simulink model "controlAerobi"  (R2017b)
settings: Solver=FixedStepDiscrete  StartTime=0.0  StopTime=inf  FixedStep=Ts  RelTol=1e-3
InitFcn:
  | load Navio2_bus;
  | Ts=0.0025;
StopFcn:
  | %save_system('controlAerobi.slx');
  | %run('D:\Eclipse_Workspaces\workspace_rasp\AutoPilot\contAerobi\UpdateFiles\CopyBuildFiles.m');
undefined symbols (not defined in the file or in its folder): DiscIntNeverNeededParam
libraries: simulink x36, sharedutil x1, sharedtransform x1, dspsigops x1
(part 1 of 4)
CloseFcn:
  | %save_system('controlAerobi.slx');
settings Model: SimulationMode=external  ExtModeTrigDuration=400000  ExtModeArchiveFileName=apAerobi  ExtModeArchiveDirName=/home/ae-grvc/Documentos/Workspace/AutoPilot/GRVCAutopilot/Logs  ExtModeLogAll=off  Creator=GRVC  LastModifiedBy=root
settings SolverCC: PositivePriorityOrder=on
settings DataIOCC: SaveFormat=Array  SaveOutput=off  SaveTime=off
settings OptimizationCC: MemcpyThreshold=128  EfficientFloat2IntCast=on  MaxStackSize=128
settings DebuggingCC: SolverPrmCheckMsg=warning  IntegerOverflowMsg=none  ParameterTunabilityLossMsg=error  InvalidFcnCallConnMsg=warning  FcnCallInpInsideContextMsg=warning  BusObjectLabelMismatch=error  RootOutportRequireBusObject=error  ModelReferenceIOMsg=error  ModelReferenceIOMismatchMessage=error  ModelReferenceDataLoggingMessage=error  StateNameClashWarn=warning  SFUnexpectedBacktrackingDiag=warning  SFNoUnconditionalDefaultTransitionDiag=warning  SFExecutionAtInitializationDiag=none  IntegerSaturationMsg=none
settings HardwareCC: ProdBitPerPointer=32  ProdBitPerSizeT=32  ProdBitPerPtrDiffT=32  ProdLargestAtomicInteger=Long  ProdLargestAtomicFloat=Double  ProdWordSize=32  ProdHWDeviceType=ARM Compatible->ARM Cortex
settings ModelReferenceCC: ModelReferenceNumInstancesAllowed=Single  ModelReferencePassRootInputsByReference=off  PropagateSignalLabelsOutOfModel=off
settings SFSimCC: SimParseCustomCode=off  MATLABDynamicMemAlloc=off
settings RTWCC: SystemTargetFile=ert.tlc  HardwareBoard=Raspberry Pi  TemplateMakefile=ert_default_tmf  GenerateReport=on  RTWVerbose=off  CustomInclude=/home/ae-grvc/Documentos/Workspace/libshm_navio  Toolchain=GNU GCC Raspberry Pi  BuildConfiguration=Faster Runs  IncludeHyperlinkInReport=on  TargetLang=C++  GenerateTraceInfo=on  GenerateTraceReport=on  GenerateTraceReportSl=on  GenerateTraceReportSf=on  GenerateTraceReportEml=on
settings RTWCC: CustomHeaderCode=|
  | #include <shm_util.h>
  | #include <shm_channels.h>
settings CodeAppCC: ForceParamTrailComments=on  IgnoreCustomStorageClasses=off  CustomSymbolStrType=$N$R$M  StateflowObjectComments=on  InternalIdentifier=Classic
settings ERTTargetCC: UtilityFuncGeneration=Shared location  MatFileLogging=on  SupportComplex=off  SupportVariableSizeSignals=on  ExtMode=on  ExtModeMexArgs='navioAE-1.local' 0 17725 5  ConvertIfToSwitch=off  SuppressUnreachableDefaultCases=off  EnableUserReplacementTypes=on  MemSecPackage=Simulink  MemSecDataConstants=MemConst

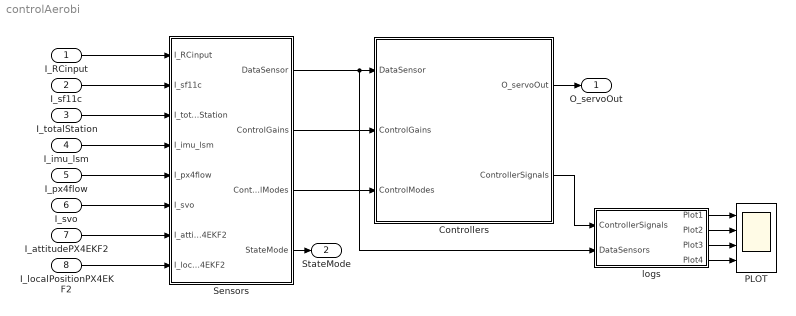
== system controlAerobi ==
  I_RCinput : Inport  OutDataTypeStr=Bus: shm_RCin
  I_sf11c : Inport  Port=2  OutDataTypeStr=Bus: shm_lightware
  I_totalStation : Inport  Port=3  OutDataTypeStr=Bus: shm_totalStation
  I_imu_lsm : Inport  Port=4  OutDataTypeStr=Bus: shm_imu
  I_px4flow : Inport  Port=5  OutDataTypeStr=Bus: shm_px4flow
  I_svo : Inport  Port=6  OutDataTypeStr=Bus: shm_svo
  I_attitudePX4EKF2 : Inport  Port=7  OutDataTypeStr=Bus: shm_attitudePX4EKF2
  I_localPositionPX4EKF2 : Inport  Port=8  OutDataTypeStr=Bus: shm_localPositionPX4EKF2
  Controllers : Subsystem
  PLOT : Scope  NumInputPorts=4
  Sensors : Subsystem
  logs : Subsystem  mask(Select signals to plot){SelectPlot1=roll, SelectPlot2=pitch, SelectPlot3=yaw, SelectPlot4=dyaw}
      mask prompts: SelectPlot1 "Select First Plot"; SelectPlot2 "Select Second Plot"; SelectPlot3 "Select Third Plot"; SelectPlot4 "Select Fourth Plot"
      mask TypeOptions SelectPlot1: roll | pitch | yaw | droll | dpitch | dyaw | x | y | z | dx | dy | dz | Rotors 1 & 2 | Rotors 3 & 4
      mask TypeOptions SelectPlot2: roll | pitch | yaw | droll | dpitch | dyaw | x | y | z | dx | dy | dz | Rotors 1 & 2 | Rotors 3 & 4
      mask TypeOptions SelectPlot3: roll | pitch | yaw | droll | dpitch | dyaw | x | y | z | dx | dy | dz | Rotors 1 & 2 | Rotors 3 & 4
      mask TypeOptions SelectPlot4: roll | pitch | yaw | droll | dpitch | dyaw | x | y | z | dx | dy | dz | Rotors 1 & 2 | Rotors 3 & 4
  O_servoOut : Outport  OutDataTypeStr=Bus: shm_RCou
  StateMode : Outport  Port=2
  wires:
  Sensors/2(ControlGains) -> Controllers/2(ControlGains)
  Sensors/3(ControlModes) -> Controllers/3(ControlModes)
  Controllers/1(O_servoOut) -> O_servoOut/1
  I_imu_lsm/1 -> Sensors/4(I_imu_lsm)
  logs/3(Plot3) -> PLOT/3
  I_px4flow/1 -> Sensors/5(I_px4flow)
  logs/4(Plot4) -> PLOT/4
  I_totalStation/1 -> Sensors/3(I_totalStation)
  logs/2(Plot2) -> PLOT/2
  Sensors/1(DataSensor) -> logs/2(DataSensors), Controllers/1(DataSensor)
  I_sf11c/1 -> Sensors/2(I_sf11c)
  Controllers/2(ControllerSignals) -> logs/1(ControllerSignals)
  Sensors/4(StateMode) -> StateMode/1
  logs/1(Plot1) -> PLOT/1
  I_RCinput/1 -> Sensors/1(I_RCinput)
  I_svo/1 -> Sensors/6(I_svo)
  I_attitudePX4EKF2/1 -> Sensors/7(I_attitudePX4EKF2)
  I_localPositionPX4EKF2/1 -> Sensors/8(I_localPositionPX4EKF2)

== system controlAerobi/Controllers ==
  DataSensor : Inport
  ControlGains : Inport  Port=2
  ControlModes : Inport  Port=3
  Quadrotor_Controllers : Subsystem
  O_servoOut : Outport  OutDataTypeStr=Bus: shm_RCou
  ControllerSignals : Outport  Port=2
  wires:
  DataSensor/1 -> Quadrotor_Controllers/1(DataSensor)
  Quadrotor_Controllers/1(ControllerSignals) -> ControllerSignals/1
  Quadrotor_Controllers/2(O_servoOut) -> O_servoOut/1
  ControlModes/1 -> Quadrotor_Controllers/3(ControlModes)
  ControlGains/1 -> Quadrotor_Controllers/2(ControlGains)

== system controlAerobi/Sensors ==
  I_RCinput : Inport  OutDataTypeStr=Bus: shm_RCin
  I_sf11c : Inport  Port=2  OutDataTypeStr=Bus: shm_lightware
  I_totalStation : Inport  Port=3  OutDataTypeStr=Bus: shm_totalStation
  I_imu_lsm : Inport  Port=4  OutDataTypeStr=Bus: shm_imu
  I_px4flow : Inport  Port=5  OutDataTypeStr=Bus: shm_px4flow
  I_svo : Inport  Port=6  OutDataTypeStr=Bus: shm_svo
  I_attitudePX4EKF2 : Inport  Port=7  OutDataTypeStr=Bus: shm_attitudePX4EKF2
  I_localPositionPX4EKF2 : Inport  Port=8  OutDataTypeStr=Bus: shm_localPositionPX4EKF2
  Bus Creator : BusCreator  Inputs=3
  Bus Creator1 : BusCreator  Inputs=2
  Geometric_Control_gains : Subsystem
  PID_cascade_gains : Subsystem
  RadioChannels : Subsystem
  ViewFlightMode : Subsystem
  attitude : Subsystem
  control_modes : Subsystem
  position : Subsystem
  DataSensor : Outport
  ControlGains : Outport  Port=2
  ControlModes : Outport  Port=3
  StateMode : Outport  Port=4
  wires:
  position/1(position_) -> Bus Creator/2  "position_"
  RadioChannels/1(Channels) -> Bus Creator/3  "channels"
  attitude/1(attitude_) -> position/1(attitude_), Bus Creator/1  "attitude_"
  I_RCinput/1 -> RadioChannels/1(I_RCinput)
  I_sf11c/1 -> position/2(I_sf11c)
  I_totalStation/1 -> position/3(I_totalStation)
  I_imu_lsm/1 -> attitude/1(I_imu_lsm)
  Bus Creator/1 -> control_modes/1(DataSensors), DataSensor/1
  PID_cascade_gains/1(PIDControlGains) -> Bus Creator1/1  "PIDgains"
  Geometric_Control_gains/1(GeometricControlGains) -> Bus Creator1/2  "GeometricGains"
  Bus Creator1/1 -> ControlGains/1
  control_modes/1(controlModes) -> position/6(ControlModes), ViewFlightMode/1(ControlModes), ControlModes/1
  ViewFlightMode/1(StateMode) -> StateMode/1
  I_px4flow/1 -> position/4(I_px4flow)
  I_svo/1 -> position/5(I_svo)
  I_attitudePX4EKF2/1 -> attitude/2(I_attitudePX4EKF2)
  I_localPositionPX4EKF2/1 -> position/7(I_localPositionPX4EKF2)

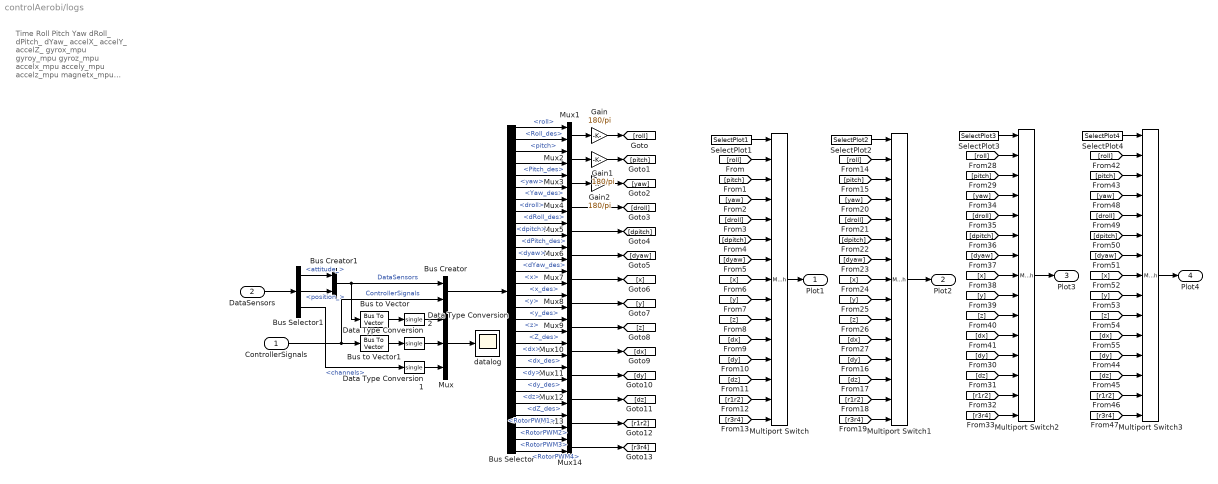
== system controlAerobi/logs ==
  note: Time
      | Roll
      | Pitch
      | Yaw
      | dRoll_
      | dPitch_
      | dYaw_
      | accelX_
      | accelY_
      | accelZ_
      | gyrox_mpu
      | gyroy_mpu
      | gyroz_mpu
      | accelx_mpu
      | accely_mpu
      | accelz_mpu
      | magnetx_mpu
      | magnety_mpu
      | magentz_mpu
      | gyrox_lsm
      | gyroy_lsm
      | gyroz_lsm
      | accelx_lsm
      | accely_lsm
      | accelz_lsm
      | magnetx_lsm
      | magnety_lsm
      | magnetz_lsm
      | GPS_solution
      | x_
      | y_
      | z_
      | dx_
      | dy_
      | dz_
      | z_sf11c
      | x_totalStation
      | y_totalStation
      | z_totalStation
      | time_totalStation
      | x_des
      | y_des
      | dx_des
      | dy_des
      | thrust
      | z_des
      | dz_des
      | roll_des
      | pitch_des
      | yaw_des
      | droll_des
      | dpitch_des
      | dyaw_des
      | RotorPWM1
      | RotorPWM2
      | RotorPWM3
      | RotorPWM4
      | Channel1
      | Channel2
      | Channel3
      | Channel4
      | Channel5
      | Channel6
      | Channel7
      | Channel8
      | Channel9
      | Channel10
  ControllerSignals : Inport
  DataSensors : Inport  Port=2
  Bus Creator : BusCreator  Inputs=2
  Bus Creator1 : BusCreator  Inputs=2
  Bus Selector : BusSelector  OutputSignals=DataSensors.attitude_.AngularPosition.roll,ControllerSignals.ControllersSignalsDesired.AttitudeSignals.AngularPositionDes.Roll_des,DataSensors.attitude_.AngularPosition.pitch,ControllerSignals.ControllersSignalsDesired.AttitudeSignals.AngularPositionDes.Pitch_des,DataSensors.attitude_.AngularPosition.yaw,ControllerSignals.ControllersSignalsDesired.AttitudeSignals.AngularPositionDes.Yaw_des,DataSensors.attitude_.AngularRates.droll,ControllerSignals.ControllersSignalsDesired.AttitudeSignals.AngularRateDes.dRoll_des,DataSensors.attitude_.AngularRates.dpitch,ControllerSignals.ControllersSignalsDesired.AttitudeSignals.AngularRateDes.dPitch_des,DataSensors.attitude_.AngularRates.dyaw,ControllerSignals.ControllersSignalsDesired.AttitudeSignals.AngularRateDes.dYaw_des,DataSensors.position_.Position.x,ControllerSignals.ControllersSignalsDesired.PositionSignals.x_des,DataSensors.position_.Position.y,ControllerSignals.ControllersSignalsDesired.PositionSignals.y_des,DataSensors.position_.Position.z,ControllerSignals.ControllersSignalsDesired.AltitudeSignals.ZController.Z_des,DataSensors.position_.Velocity.dx,ControllerSignals.ControllersSignalsDesired.PositionSignals.dx_des,DataSensors.position_.Velocity.dy,ControllerSignals.ControllersSignalsDesired.PositionSignals.dy_des,DataSensors.position_.Velocity.dz,ControllerSignals.ControllersSignalsDesired.AltitudeSignals.ZController.dZ_des,ControllerSignals.MixerSignals.RotorPWMSignals.RotorPWM1,ControllerSignals.MixerSignals.RotorPWMSignals.RotorPWM2,ControllerSignals.MixerSignals.RotorPWMSignals.RotorPWM3,ControllerSignals.MixerSignals.RotorPWMSignals.RotorPWM4
  Bus Selector1 : BusSelector  OutputSignals=attitude_,position_,channels
  Bus to Vector : BusToVector
  Bus to Vector1 : BusToVector
  Data Type Conversion : DataTypeConversion  OutDataTypeStr=single
  Data Type Conversion1 : DataTypeConversion  OutDataTypeStr=single
  Data Type Conversion2 : DataTypeConversion  OutDataTypeStr=single
  Gain : Gain  Gain=180/pi
  Gain1 : Gain  Gain=180/pi
  Gain2 : Gain  Gain=180/pi
  Multiport Switch{,1..3} (4 alike) : MultiPortSwitch  Inputs=14
  Mux : Mux  Inputs=3
  Mux{1..14} (14 alike) : Mux  Inputs=2
  SelectPlot1 : Constant  Value=SelectPlot1
  SelectPlot2 : Constant  Value=SelectPlot2
  SelectPlot3 : Constant  Value=SelectPlot3
  SelectPlot4 : Constant  Value=SelectPlot4
  datalog : Scope
  Plot1 : Outport
  Plot2 : Outport  Port=2
  Plot3 : Outport  Port=3
  Plot4 : Outport  Port=4
  wires:
  ControllerSignals/1 -> Bus to Vector1/1, Bus Creator/2  "ControllerSignals"
  Mux/1 -> datalog/1
  Bus to Vector1/1 -> Data Type Conversion/1
  Bus Creator/1 -> Bus Selector/1
  Bus Selector/2 -> Mux1/2  "<Roll_des>"
  Bus Selector/1 -> Mux1/1  "<roll>"
  Bus Selector/3 -> Mux2/1  "<pitch>"
  Bus Selector/4 -> Mux2/2  "<Pitch_des>"
  Bus Selector/5 -> Mux3/1  "<yaw>"
  Bus Selector/6 -> Mux3/2  "<Yaw_des>"
  Bus Selector/8 -> Mux4/2  "<dRoll_des>"
  Bus Selector/7 -> Mux4/1  "<droll>"
  Bus Selector/9 -> Mux5/1  "<dpitch>"
  Bus Selector/10 -> Mux5/2  "<dPitch_des>"
  Bus Selector/12 -> Mux6/2  "<dYaw_des>"
  Bus Selector/11 -> Mux6/1  "<dyaw>"
  Bus Selector/13 -> Mux7/1  "<x>"
  Bus Selector/14 -> Mux7/2  "<x_des>"
  Bus Selector/15 -> Mux8/1  "<y>"
  Bus Selector/16 -> Mux8/2  "<y_des>"
  Bus Selector/17 -> Mux9/1  "<z>"
  Bus Selector/18 -> Mux9/2  "<Z_des>"
  Bus Selector/19 -> Mux10/1  "<dx>"
  Bus Selector/20 -> Mux10/2  "<dx_des>"
  Bus Selector/22 -> Mux11/2  "<dy_des>"
  Bus Selector/21 -> Mux11/1  "<dy>"
  Bus Selector/23 -> Mux12/1  "<dz>"
  Bus Selector/24 -> Mux12/2  "<dZ_des>"
  Bus Selector/25 -> Mux13/1  "<RotorPWM1>"
  Bus Selector/26 -> Mux13/2  "<RotorPWM2>"
  Bus Selector/27 -> Mux14/1  "<RotorPWM3>"
  Bus Selector/28 -> Mux14/2  "<RotorPWM4>"
  SelectPlot1/1 -> Multiport Switch/1
  Mux2/1 -> Gain1/1
  Mux3/1 -> Gain2/1
  Mux4/1 -> [droll]
  Mux5/1 -> [dpitch]
  Mux6/1 -> [dyaw]
  Mux7/1 -> [x]
  Mux8/1 -> [y]
  Mux9/1 -> [z]
  Mux10/1 -> [dx]
  Mux11/1 -> [dy]
  Mux12/1 -> [dz]
  [y] -> Multiport Switch/9
  [x] -> Multiport Switch/8
  [dpitch] -> Multiport Switch/6
  [dyaw] -> Multiport Switch/7
  [z] -> Multiport Switch/10
  [droll] -> Multiport Switch/5
  [dx] -> Multiport Switch/11
  [yaw] -> Multiport Switch/4
  [pitch] -> Multiport Switch/3
  [dz] -> Multiport Switch/13
  [dy] -> Multiport Switch/12
  [roll] -> Multiport Switch/2
  [r1r2] -> Multiport Switch/14
  [r3r4] -> Multiport Switch/15
  SelectPlot2/1 -> Multiport Switch1/1
  [y] -> Multiport Switch1/9
  [x] -> Multiport Switch1/8
  [dpitch] -> Multiport Switch1/6
  [dyaw] -> Multiport Switch1/7
  [z] -> Multiport Switch1/10
  [droll] -> Multiport Switch1/5
  [dx] -> Multiport Switch1/11
  [yaw] -> Multiport Switch1/4
  [pitch] -> Multiport Switch1/3
  [dz] -> Multiport Switch1/13
  [dy] -> Multiport Switch1/12
  [roll] -> Multiport Switch1/2
  [r1r2] -> Multiport Switch1/14
  [r3r4] -> Multiport Switch1/15
  SelectPlot3/1 -> Multiport Switch2/1
  [y] -> Multiport Switch2/9
  [x] -> Multiport Switch2/8
  [dpitch] -> Multiport Switch2/6
  [dyaw] -> Multiport Switch2/7
  [z] -> Multiport Switch2/10
  [droll] -> Multiport Switch2/5
  [dx] -> Multiport Switch2/11
  [yaw] -> Multiport Switch2/4
  [pitch] -> Multiport Switch2/3
  [dz] -> Multiport Switch2/13
  [dy] -> Multiport Switch2/12
  [roll] -> Multiport Switch2/2
  [r1r2] -> Multiport Switch2/14
  [r3r4] -> Multiport Switch2/15
  SelectPlot4/1 -> Multiport Switch3/1
  [y] -> Multiport Switch3/9
  [x] -> Multiport Switch3/8
  [dpitch] -> Multiport Switch3/6
  [dyaw] -> Multiport Switch3/7
  [z] -> Multiport Switch3/10
  [droll] -> Multiport Switch3/5
  [dx] -> Multiport Switch3/11
  [yaw] -> Multiport Switch3/4
  [pitch] -> Multiport Switch3/3
  [dz] -> Multiport Switch3/13
  [dy] -> Multiport Switch3/12
  [roll] -> Multiport Switch3/2
  [r1r2] -> Multiport Switch3/14
  [r3r4] -> Multiport Switch3/15
  Multiport Switch/1 -> Plot1/1
  Multiport Switch1/1 -> Plot2/1
  Multiport Switch2/1 -> Plot3/1
  Multiport Switch3/1 -> Plot4/1
  Mux1/1 -> Gain/1
  Gain/1 -> [roll]
  Gain1/1 -> [pitch]
  Gain2/1 -> [yaw]
  Data Type Conversion/1 -> Mux/2
  Bus to Vector/1 -> Data Type Conversion2/1
  Mux13/1 -> [r1r2]
  Mux14/1 -> [r3r4]
  DataSensors/1 -> Bus Selector1/1
  Bus Creator1/1 -> Bus to Vector/1, Bus Creator/1  "DataSensors"
  Bus Selector1/1 -> Bus Creator1/1  "<attitude_>"
  Bus Selector1/2 -> Bus Creator1/2  "<position_>"
  Bus Selector1/3 -> Data Type Conversion1/1  "<channels>"
  Data Type Conversion1/1 -> Mux/3
  Data Type Conversion2/1 -> Mux/1

== system controlAerobi/Controllers/Quadrotor_Controllers ==
  DataSensor : Inport
  ControlGains : Inport  Port=2
  ControlModes : Inport  Port=3
  Bus Creator : BusCreator  Inputs=2
  Geometric_controller : Subsystem
  PID_cascade_controllers : Subsystem
  mixer : Subsystem
  switch_controllers : Subsystem
  ControllerSignals : Outport
  O_servoOut : Outport  Port=2  OutDataTypeStr=Bus: shm_RCou
  wires:
  mixer/2(O_servoOut) -> O_servoOut/1
  Bus Creator/1 -> ControllerSignals/1
  mixer/1(MixerSignals) -> Bus Creator/2  "MixerSignals"
  ControlModes/1 -> switch_controllers/3(ControlModes), mixer/2(ControlModes), Geometric_controller/3(ControlModes), PID_cascade_controllers/2(ControlModes)
  DataSensor/1 -> Geometric_controller/1(DataSensor), PID_cascade_controllers/1(DataSensor)
  ControlGains/1 -> Geometric_controller/2(ControlGains), PID_cascade_controllers/3(ControlGains)
  PID_cascade_controllers/1(ControllersSignalsDesired) -> Bus Creator/1  "ControllersSignalsDesired"
  PID_cascade_controllers/2(U_PID) -> switch_controllers/1(U_PID)
  Geometric_controller/1(U_GeometricControl) -> switch_controllers/2(U_GeometricControl)
  switch_controllers/1(U) -> mixer/1(U)

== system controlAerobi/Sensors/Geometric_Control_gains ==
  Bus Creator1 : BusCreator  Inputs=4
  Bus Creator2 : BusCreator  Inputs=10
  Bus Creator3 : BusCreator  Inputs=2
  CTf : Constant  Value=0.0008
  J : Constant  Value=[0.08 0 0; 0 0.08 0; 0 0 0.14]
  Mass : Constant  Value=1.97
  c1 : Constant  Value=[0.8; 0.8; 0.8]
  c2 : Constant  Value=[3; 3; 3]
  d : Constant  Value=0.2675
  k_I : Constant  Value=[55; 55; 55]
  k_Omega : Constant  Value=[8; 8; 8]
  k_R : Constant  Value=[60; 60; 60]
  k_i : Constant  Value=[0; 0; 0]
  k_v : Constant  Value=[10; 10; 10]
  k_x : Constant  Value=[10; 10; 10]
  sat_P : Constant  Value=[inf; inf; inf]
  sat_R : Constant  Value=[inf; inf; inf]
  GeometricControlGains : Outport
  wires:
  J/1 -> Bus Creator1/1  "J"
  CTf/1 -> Bus Creator1/4  "CTf"
  Mass/1 -> Bus Creator1/2  "Mass"
  d/1 -> Bus Creator1/3  "d"
  Bus Creator1/1 -> Bus Creator3/1  "UAVparameters"
  Bus Creator2/1 -> Bus Creator3/2  "Gains"
  Bus Creator3/1 -> GeometricControlGains/1
  k_R/1 -> Bus Creator2/1  "k_R"
  k_Omega/1 -> Bus Creator2/2  "k_Omega"
  k_x/1 -> Bus Creator2/6  "k_x"
  k_v/1 -> Bus Creator2/7  "k_v"
  c2/1 -> Bus Creator2/4  "c2"
  sat_R/1 -> Bus Creator2/5  "sat_R"
  k_I/1 -> Bus Creator2/3  "k_I"
  k_i/1 -> Bus Creator2/8  "k_i"
  c1/1 -> Bus Creator2/9  "c1"
  sat_P/1 -> Bus Creator2/10  "sat_P"

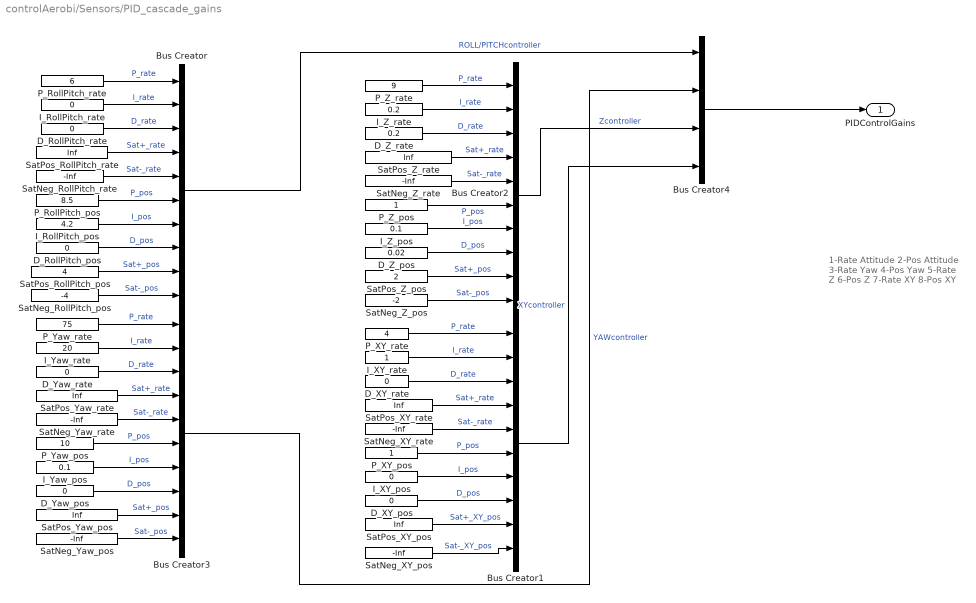
== system controlAerobi/Sensors/PID_cascade_gains ==
  note: 1-Rate Attitude
      | 2-Pos Attitude
      | 3-Rate Yaw
      | 4-Pos Yaw
      | 5-Rate Z
      | 6-Pos Z
      | 7-Rate XY
      | 8-Pos XY
  Bus Creator{,1..3} (4 alike) : BusCreator  Inputs=10
  Bus Creator4 : BusCreator  Inputs=4
  D_RollPitch_pos : Constant  Value=0
  D_RollPitch_rate : Constant  Value=0
  D_XY_pos : Constant  Value=0
  D_XY_rate : Constant  Value=0
  D_Yaw_pos : Constant  Value=0
  D_Yaw_rate : Constant  Value=0
  D_Z_pos : Constant  Value=0.02
  D_Z_rate : Constant  Value=0.2
  I_RollPitch_pos : Constant  Value=4.2
  I_RollPitch_rate : Constant  Value=0
  I_XY_pos : Constant  Value=0
  I_XY_rate : Constant
  I_Yaw_pos : Constant  Value=0.1
  I_Yaw_rate : Constant  Value=20
  I_Z_pos : Constant  Value=0.1
  I_Z_rate : Constant  Value=0.2
  P_RollPitch_pos : Constant  Value=8.5
  P_RollPitch_rate : Constant  Value=6
  P_XY_pos : Constant
  P_XY_rate : Constant  Value=4
  P_Yaw_pos : Constant  Value=10
  P_Yaw_rate : Constant  Value=75
  P_Z_pos : Constant
  P_Z_rate : Constant  Value=9
  SatNeg_RollPitch_pos : Constant  Value=-4
  SatNeg_RollPitch_rate : Constant  Value=-Inf
  SatNeg_XY_pos : Constant  Value=-Inf
  SatNeg_XY_rate : Constant  Value=-Inf
  SatNeg_Yaw_pos : Constant  Value=-Inf
  SatNeg_Yaw_rate : Constant  Value=-Inf
  SatNeg_Z_pos : Constant  Value=-2
  SatNeg_Z_rate : Constant  Value=-Inf
  SatPos_RollPitch_pos : Constant  Value=4
  SatPos_RollPitch_rate : Constant  Value=Inf
  SatPos_XY_pos : Constant  Value=Inf
  SatPos_XY_rate : Constant  Value=Inf
  SatPos_Yaw_pos : Constant  Value=Inf
  SatPos_Yaw_rate : Constant  Value=Inf
  SatPos_Z_pos : Constant  Value=2
  SatPos_Z_rate : Constant  Value=Inf
  PIDControlGains : Outport
  wires:
  SatPos_RollPitch_rate/1 -> Bus Creator/4  "Sat+_rate"
  D_RollPitch_rate/1 -> Bus Creator/3  "D_rate"
  P_RollPitch_rate/1 -> Bus Creator/1  "P_rate"
  I_RollPitch_rate/1 -> Bus Creator/2  "I_rate"
  SatNeg_RollPitch_rate/1 -> Bus Creator/5  "Sat-_rate"
  D_RollPitch_pos/1 -> Bus Creator/8  "D_pos"
  I_RollPitch_pos/1 -> Bus Creator/7  "I_pos"
  P_RollPitch_pos/1 -> Bus Creator/6  "P_pos"
  SatNeg_RollPitch_pos/1 -> Bus Creator/10  "Sat-_pos"
  SatPos_RollPitch_pos/1 -> Bus Creator/9  "Sat+_pos"
  SatPos_Yaw_rate/1 -> Bus Creator3/4  "Sat+_rate"
  SatNeg_Yaw_rate/1 -> Bus Creator3/5  "Sat-_rate"
  P_Yaw_rate/1 -> Bus Creator3/1  "P_rate"
  I_Yaw_rate/1 -> Bus Creator3/2  "I_rate"
  D_Yaw_rate/1 -> Bus Creator3/3  "D_rate"
  P_Yaw_pos/1 -> Bus Creator3/6  "P_pos"
  SatPos_Yaw_pos/1 -> Bus Creator3/9  "Sat+_pos"
  I_Yaw_pos/1 -> Bus Creator3/7  "I_pos"
  SatNeg_Yaw_pos/1 -> Bus Creator3/10  "Sat-_pos"
  D_Yaw_pos/1 -> Bus Creator3/8  "D_pos"
  SatPos_Z_rate/1 -> Bus Creator2/4  "Sat+_rate"
  SatNeg_Z_rate/1 -> Bus Creator2/5  "Sat-_rate"
  D_Z_rate/1 -> Bus Creator2/3  "D_rate"
  I_Z_rate/1 -> Bus Creator2/2  "I_rate"
  P_Z_rate/1 -> Bus Creator2/1  "P_rate"
  P_Z_pos/1 -> Bus Creator2/6  "P_pos"
  I_Z_pos/1 -> Bus Creator2/7  "I_pos"
  D_Z_pos/1 -> Bus Creator2/8  "D_pos"
  SatPos_Z_pos/1 -> Bus Creator2/9  "Sat+_pos"
  SatNeg_Z_pos/1 -> Bus Creator2/10  "Sat-_pos"
  SatPos_XY_rate/1 -> Bus Creator1/4  "Sat+_rate"
  SatNeg_XY_rate/1 -> Bus Creator1/5  "Sat-_rate"
  I_XY_rate/1 -> Bus Creator1/2  "I_rate"
  D_XY_rate/1 -> Bus Creator1/3  "D_rate"
  P_XY_rate/1 -> Bus Creator1/1  "P_rate"
  P_XY_pos/1 -> Bus Creator1/6  "P_pos"
  SatPos_XY_pos/1 -> Bus Creator1/9  "Sat+_XY_pos"
  SatNeg_XY_pos/1 -> Bus Creator1/10  "Sat-_XY_pos"
  I_XY_pos/1 -> Bus Creator1/7  "I_pos"
  Bus Creator/1 -> Bus Creator4/1  "ROLL/PITCHcontroller"
  Bus Creator3/1 -> Bus Creator4/2  "YAWcontroller"
  Bus Creator2/1 -> Bus Creator4/3  "Zcontroller"
  Bus Creator1/1 -> Bus Creator4/4  "XYcontroller"
  Bus Creator4/1 -> PIDControlGains/1
  D_XY_pos/1 -> Bus Creator1/8  "D_pos"

== system controlAerobi/Sensors/RadioChannels ==
  I_RCinput : Inport  OutDataTypeStr=Bus: shm_RCin
  Bus Selector2 : BusSelector  OutputSignals=_channel1,_channel2,_channel3,_channel4,_channel5,_channel6,_channel7,_channel8,_channel9,_channel10
  Mux1 : Mux  Inputs=10
  Channels : Outport
  wires:
  Bus Selector2/3 -> Mux1/3  "<_channel3>"
  Bus Selector2/4 -> Mux1/4  "<_channel4>"
  Bus Selector2/2 -> Mux1/2  "<_channel2>"
  Bus Selector2/5 -> Mux1/5  "<_channel5>"
  Bus Selector2/10 -> Mux1/10  "<_channel10>"
  Bus Selector2/1 -> Mux1/1  "<_channel1>"
  Bus Selector2/6 -> Mux1/6  "<_channel6>"
  Bus Selector2/7 -> Mux1/7  "<_channel7>"
  Bus Selector2/8 -> Mux1/8  "<_channel8>"
  Bus Selector2/9 -> Mux1/9  "<_channel9>"
  Mux1/1 -> Channels/1
  I_RCinput/1 -> Bus Selector2/1

== system controlAerobi/Sensors/ViewFlightMode ==
  ControlModes : Inport
  Bus Selector1 : BusSelector  OutputSignals=ModeControl.RESET,ModeControl.ALTHOLD,ModeControl.POS_HOLD
  Mux1 : Mux  Inputs=3
  State : Display
  StateMode : Outport
  wires:
  ControlModes/1 -> Bus Selector1/1
  Bus Selector1/2 -> Mux1/2  "<ALTHOLD>"
  Mux1/1 -> StateMode/1, State/1
  Bus Selector1/1 -> Mux1/1  "<RESET>"
  Bus Selector1/3 -> Mux1/3  "<POS_HOLD>"

== system controlAerobi/Sensors/attitude ==
  I_imu_lsm : Inport  OutDataTypeStr=Bus: shm_imu
  I_attitudePX4EKF2 : Inport  Port=2  OutDataTypeStr=Bus: shm_attitudePX4EKF2
  AttitudeEstimator : Subsystem
  Bus Creator2 : BusCreator  Inputs=4
  attitude_ : Outport
  wires:
  AttitudeEstimator/2(AnguraRates) -> Bus Creator2/2  "AngularRates"
  Bus Creator2/1 -> attitude_/1
  AttitudeEstimator/1(Attitude) -> Bus Creator2/1  "AngularPosition"
  AttitudeEstimator/3(Accelerometer) -> Bus Creator2/3  "Accelerometer"
  AttitudeEstimator/4(imuRaw) -> Bus Creator2/4  "imuRaw"
  I_imu_lsm/1 -> AttitudeEstimator/1(I_imu_lsm)
  I_attitudePX4EKF2/1 -> AttitudeEstimator/2(I_attitudePX4EKF2)

== system controlAerobi/Sensors/control_modes ==
  note: MODE:
      | 1.-ATTITUDE/RATE
      | 2.-ALT. HOLD
      | 3.-POS. HOLD
  DataSensors : Inport
  Bus Creator2 : BusCreator  Inputs=3
  ModeBlock : Subsystem
  PositionDesired : Subsystem
  Signals_to_references : Subsystem
  controlModes : Outport
  wires:
  Bus Creator2/1 -> controlModes/1
  DataSensors/1 -> Signals_to_references/1(uiPilotChannels), ModeBlock/1(Sticks)
  Signals_to_references/1(RemoteControl) -> Bus Creator2/1  "RemoteControl"
  ModeBlock/1(ModeControl) -> Bus Creator2/2  "ModeControl"
  PositionDesired/1(PositionDesired) -> Bus Creator2/3  "PositionDesired"

== system controlAerobi/Sensors/position ==
  attitude_ : Inport
  I_sf11c : Inport  Port=2  OutDataTypeStr=Bus: shm_lightware
  I_totalStation : Inport  Port=3  OutDataTypeStr=Bus: shm_totalStation
  I_px4flow : Inport  Port=4  OutDataTypeStr=Bus: shm_px4flow
  I_svo : Inport  Port=5  OutDataTypeStr=Bus: shm_svo
  ControlModes : Inport  Port=6
  I_localPositionPX4EKF2 : Inport  Port=7  OutDataTypeStr=Bus: shm_localPositionPX4EKF2
  Bus Creator2 : BusCreator  Inputs=4
  EKF_total_Station_Lidar : Subsystem
  GPS_px4 : Subsystem
  KQ : Constant  Value="[ 0 0.005  0 0.005  0 0.0025]"
  KR : Constant  Value=[0.01 0.1 0.01 0.1 0.05]
  PX4 : Scope
  SVO : Scope
  d_prism : Constant  Value=0.105
  d_sf11 : Constant  Value=0.048
  px4fow : Subsystem
  selector : Subsystem
  svo : Subsystem
  position_ : Outport
  wires:
  selector/1(GPS_Solution) -> Bus Creator2/1  "GPS_Solution"
  Bus Creator2/1 -> position_/1
  I_totalStation/1 -> EKF_total_Station_Lidar/1(I_totalStation), selector/1(I_totalStation)
  I_sf11c/1 -> EKF_total_Station_Lidar/2(I_sf11c)
  attitude_/1 -> EKF_total_Station_Lidar/3(attitude_), px4fow/1(attitude_)
  d_sf11/1 -> EKF_total_Station_Lidar/4(d_sf11)
  d_prism/1 -> EKF_total_Station_Lidar/5(d_prism)
  KQ/1 -> EKF_total_Station_Lidar/6(KQ)
  KR/1 -> EKF_total_Station_Lidar/7(KR)
  EKF_total_Station_Lidar/3(posRaw) -> Bus Creator2/4  "posRaw"
  selector/2(Position) -> Bus Creator2/2  "Position"
  selector/3(Velocity) -> Bus Creator2/3  "Velocity"
  GPS_px4/1(NED_position) -> selector/2(NED_pos_PX4)
  GPS_px4/2(NED_speed) -> selector/3(NED_vel_PX4)
  EKF_total_Station_Lidar/1(NED_position) -> selector/4(NED_pos_EKF)
  EKF_total_Station_Lidar/2(NED_speed) -> selector/5(NED_vel_EKF)
  ControlModes/1 -> px4fow/2(ControlModes), EKF_total_Station_Lidar/8(ControlModes)
  I_px4flow/1 -> px4fow/3(I_px4flow)
  px4fow/1(dxdyaxay) -> selector/6(NED_vel_PX4FLOW), PX4/1
  I_svo/1 -> svo/1(I_svo)
  svo/1(XYZ) -> SVO/1
  I_localPositionPX4EKF2/1 -> GPS_px4/1(I_localPositionPX4EKF2)

== system controlAerobi/Controllers/Quadrotor_Controllers/Geometric_controller ==
  DataSensor : Inport
  ControlGains : Inport  Port=2
  ControlModes : Inport  Port=3
  Bus Selector2 : BusSelector  OutputSignals=ModeControl.ALTHOLD,RemoteControl.Thrust/Zdes,ModeControl.RESET
  Mux : Mux
  Reset : Constant  Value=[0;0;0;0]
  Switch : Switch  Criteria=u2 ~= 0
  Switch1 : Switch  Criteria=u2 ~= 0
  attitude_tracking : Subsystem
  trajectory_tracking : Subsystem
  U_GeometricControl : Outport
  wires:
  Switch/1 -> U_GeometricControl/1
  Mux/1 -> Switch/1
  Reset/1 -> Switch/3
  DataSensor/1 -> trajectory_tracking/1(DataSensor), attitude_tracking/2(DataSensor)
  ControlGains/1 -> trajectory_tracking/2(ControlGains), attitude_tracking/3(ControlGains)
  ControlModes/1 -> trajectory_tracking/3(ControlModes), Bus Selector2/1, attitude_tracking/4(ControlModes)
  attitude_tracking/1(U2) -> Mux/2
  attitude_tracking/2(U3) -> Mux/3
  attitude_tracking/3(U4) -> Mux/4
  Switch1/1 -> Mux/1
  trajectory_tracking/1(f) -> Switch1/1
  Bus Selector2/2 -> Switch1/3  "<Thrust/Zdes>"
  trajectory_tracking/2(R_d_tracking) -> attitude_tracking/1(R_d_tracking)
  Bus Selector2/1 -> Switch1/2  "<ALTHOLD>"
  Bus Selector2/3 -> Switch/2  "<RESET>"

== system controlAerobi/Controllers/Quadrotor_Controllers/PID_cascade_controllers ==
  DataSensor : Inport
  ControlModes : Inport  Port=2
  ControlGains : Inport  Port=3
  Bus Creator1 : BusCreator  Inputs=3
  Mux : Mux
  PID_ATTITUDE_CONTROLLER : Subsystem
  PID_POSITION_CONTROLLER : Subsystem
  ControllersSignalsDesired : Outport
  U_PID : Outport  Port=2
  wires:
  ControlModes/1 -> PID_ATTITUDE_CONTROLLER/2(ControlModes), PID_POSITION_CONTROLLER/2(ControlModes)
  ControlGains/1 -> PID_ATTITUDE_CONTROLLER/3(ControlGains), PID_POSITION_CONTROLLER/3(ControlGains)
  DataSensor/1 -> PID_POSITION_CONTROLLER/1(DataSensor), PID_ATTITUDE_CONTROLLER/1(DataSensor)
  PID_POSITION_CONTROLLER/1(ref_att) -> PID_ATTITUDE_CONTROLLER/4(ref_att)
  PID_POSITION_CONTROLLER/4(U1) -> Mux/1  "U1"
  PID_ATTITUDE_CONTROLLER/3(U4) -> Mux/4  "U4"
  PID_ATTITUDE_CONTROLLER/2(U3) -> Mux/3  "U3"
  PID_ATTITUDE_CONTROLLER/1(U2) -> Mux/2  "U2"
  Mux/1 -> U_PID/1
  PID_POSITION_CONTROLLER/2(PositionSignals) -> Bus Creator1/1  "PositionSignals"
  PID_POSITION_CONTROLLER/3(AltitudeSignals) -> Bus Creator1/2  "AltitudeSignals"
  PID_ATTITUDE_CONTROLLER/4(AttitudeSignals) -> Bus Creator1/3  "AttitudeSignals"
  Bus Creator1/1 -> ControllersSignalsDesired/1

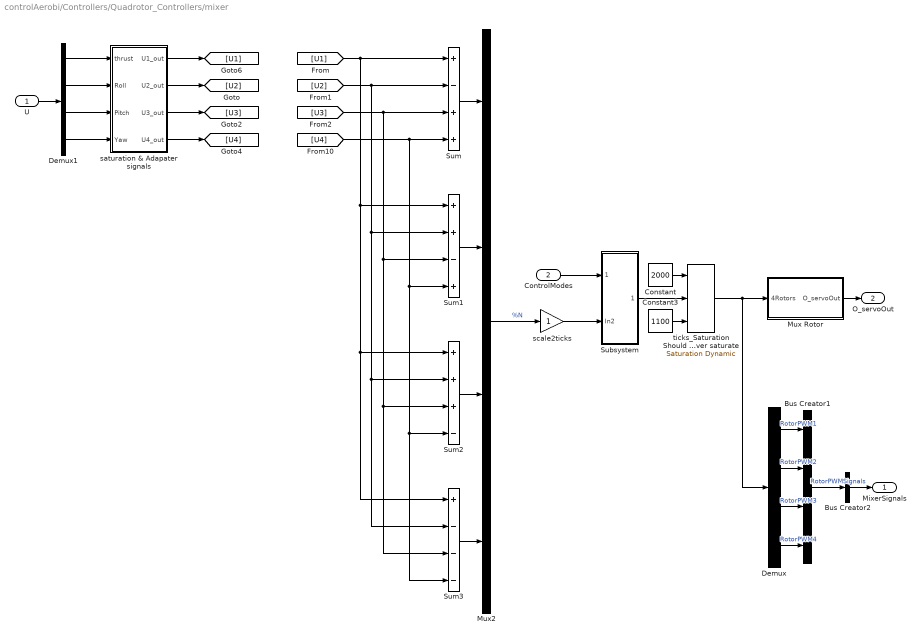
== system controlAerobi/Controllers/Quadrotor_Controllers/mixer ==
  U : Inport
  ControlModes : Inport  Port=2
  Bus Creator1 : BusCreator  Inputs=4
  Bus Creator2 : BusCreator  Inputs=1
  Constant : Constant  Value=2000
  Constant3 : Constant  Value=1100
  Demux : Demux
  Demux1 : Demux
  Mux Rotor : Subsystem
  Mux2 : Mux
  Subsystem : Subsystem
  Sum : Sum  Inputs=+-++
  Sum1 : Sum  Inputs=++-+
  Sum2 : Sum  Inputs=+++-
  Sum3 : Sum  Inputs=+---
  saturation & Adapater signals : Subsystem
  scale2ticks : Gain
  ticks_Saturation Should Never saturate : simulink/Discontinuities/Saturation Dynamic  OutMin=[]  OutMax=[]  OutDataTypeStr=Inherit: Same as second input  OutDataType=fixdt(1, 16)  OutScaling=2^-10  DoSatur=off
  MixerSignals : Outport
  O_servoOut : Outport  Port=2  OutDataTypeStr=Bus: shm_RCou
  wires:
  Constant3/1 -> ticks_Saturation Should Never saturate/3
  Constant/1 -> ticks_Saturation Should Never saturate/1
  Mux2/1 -> scale2ticks/1  "%N"
  Sum/1 -> Mux2/1
  Sum1/1 -> Mux2/2
  Sum3/1 -> Mux2/4
  ticks_Saturation Should Never saturate/1 -> Mux Rotor/1(4Rotors), Demux/1
  Sum2/1 -> Mux2/3
  saturation & Adapater signals/1(U1_out) -> [U1]
  saturation & Adapater signals/2(U2_out) -> [U2]
  saturation & Adapater signals/3(U3_out) -> [U3]
  Demux/1 -> Bus Creator1/1  "RotorPWM1"
  Demux/2 -> Bus Creator1/2  "RotorPWM2"
  Demux/3 -> Bus Creator1/3  "RotorPWM3"
  Demux/4 -> Bus Creator1/4  "RotorPWM4"
  Bus Creator1/1 -> Bus Creator2/1  "RotorPWMSignals"
  Bus Creator2/1 -> MixerSignals/1
  Mux Rotor/1(O_servoOut) -> O_servoOut/1
  ControlModes/1 -> Subsystem/1(CONTROL/MODE SIGNALS)
  Subsystem/1(Out1) -> ticks_Saturation Should Never saturate/2
  scale2ticks/1 -> Subsystem/2(In2)
  [U4] -> Sum3/4, Sum2/4, Sum1/4, Sum/4
  [U2] -> Sum1/2, Sum3/2, Sum2/2, Sum/2
  [U1] -> Sum/1, Sum1/1, Sum3/1, Sum2/1
  [U3] -> Sum3/3, Sum2/3, Sum1/3, Sum/3
  saturation & Adapater signals/4(U4_out) -> [U4]
  U/1 -> Demux1/1
  Demux1/2 -> saturation & Adapater signals/2(Roll)
  Demux1/3 -> saturation & Adapater signals/3(Pitch)
  Demux1/1 -> saturation & Adapater signals/1(thrust)
  Demux1/4 -> saturation & Adapater signals/4(Yaw)

== system controlAerobi/Controllers/Quadrotor_Controllers/switch_controllers ==
  U_PID : Inport
  U_GeometricControl : Inport  Port=2
  ControlModes : Inport  Port=3
  Bus Selector : BusSelector  OutputSignals=ModeControl.EnableGeometricControl
  Constant : Constant  Value=0  OutDataTypeStr=boolean
  Demux : Demux
  Demux1 : Demux
  Logical Operator : Logic  AllPortsSameDT=off  OutDataTypeStr=boolean
  Mux : Mux
  Switch : Switch  Criteria=u2 ~= 0
  Switch1 : Switch  Criteria=u2 ~= 0
  Switch2 : Switch  Criteria=u2 ~= 0
  Terminator1 : Terminator
  U : Outport
  wires:
  ControlModes/1 -> Bus Selector/1
  U_PID/1 -> Demux/1
  U_GeometricControl/1 -> Demux1/1
  Mux/1 -> U/1
  Bus Selector/1 -> Switch/2, Logical Operator/1, Switch1/2  "<EnableGeometricControl>"
  Switch1/1 -> Mux/3
  Switch/1 -> Mux/2
  Demux/4 -> Mux/4
  Demux1/2 -> Switch/1
  Demux1/3 -> Switch1/1
  Demux/2 -> Switch/3
  Demux/3 -> Switch1/3
  Demux1/1 -> Switch2/1
  Demux1/4 -> Terminator1/1
  Switch2/1 -> Mux/1
  Demux/1 -> Switch2/3
  Logical Operator/1 -> Switch2/2
  Constant/1 -> Logical Operator/2

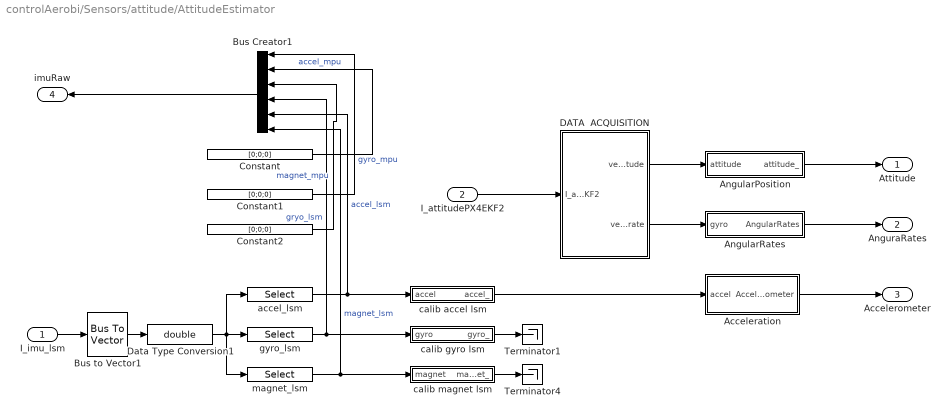
== system controlAerobi/Sensors/attitude/AttitudeEstimator ==
  I_imu_lsm : Inport  OutDataTypeStr=Bus: shm_imu
  I_attitudePX4EKF2 : Inport  Port=2  OutDataTypeStr=Bus: shm_attitudePX4EKF2
  Acceleration : Subsystem
  AngularPosition : Subsystem
  AngularRates : Subsystem
  Bus Creator1 : BusCreator  Inputs=6
  Bus to Vector1 : BusToVector
  Constant : Constant  Value=[0;0;0]
  Constant1 : Constant  Value=[0;0;0]
  Constant2 : Constant  Value=[0;0;0]
  DATA  ACQUISITION : Subsystem
  Data Type Conversion1 : DataTypeConversion  OutDataTypeStr=double
  Terminator1 : Terminator
  Terminator4 : Terminator
  accel_lsm : Selector  InputPortWidth=10  IndexOptions=Index vector (dialog)  Indices=[2 3 4]  OutputSizes=1
  calib accel lsm : Subsystem
  calib gyro lsm : Subsystem
  calib magnet lsm : Subsystem
  gyro_lsm : Selector  InputPortWidth=10  IndexOptions=Index vector (dialog)  Indices=[5 6 7]  OutputSizes=1
  magnet_lsm : Selector  InputPortWidth=10  IndexOptions=Index vector (dialog)  Indices=[8 9 10]  OutputSizes=1
  Attitude : Outport
  AnguraRates : Outport  Port=2
  Accelerometer : Outport  Port=3
  imuRaw : Outport  Port=4
  wires:
  Constant/1 -> Bus Creator1/2  "accel_mpu"
  Constant2/1 -> Bus Creator1/3  "magnet_mpu"
  Constant1/1 -> Bus Creator1/1  "gyro_mpu"
  Acceleration/1(Accelerometer) -> Accelerometer/1
  Bus Creator1/1 -> imuRaw/1
  Bus to Vector1/1 -> Data Type Conversion1/1
  Data Type Conversion1/1 -> accel_lsm/1, gyro_lsm/1, magnet_lsm/1
  I_imu_lsm/1 -> Bus to Vector1/1
  gyro_lsm/1 -> calib gyro lsm/1(gyro), Bus Creator1/4  "gryo_lsm"
  accel_lsm/1 -> calib accel lsm/1(accel), Bus Creator1/5  "accel_lsm"
  magnet_lsm/1 -> calib magnet lsm/1(magnet), Bus Creator1/6  "magnet_lsm"
  calib accel lsm/1(accel_) -> Acceleration/1(accel)
  AngularPosition/1(attitude_) -> Attitude/1
  DATA  ACQUISITION/1(vehicle_attitude) -> AngularPosition/1(attitude)
  calib magnet lsm/1(magnet_) -> Terminator4/1
  DATA  ACQUISITION/2(vehicle_attitude_rate) -> AngularRates/1(gyro)
  AngularRates/1(AngularRates) -> AnguraRates/1
  calib gyro lsm/1(gyro_) -> Terminator1/1
  I_attitudePX4EKF2/1 -> DATA  ACQUISITION/1(I_attitudePX4EKF2)

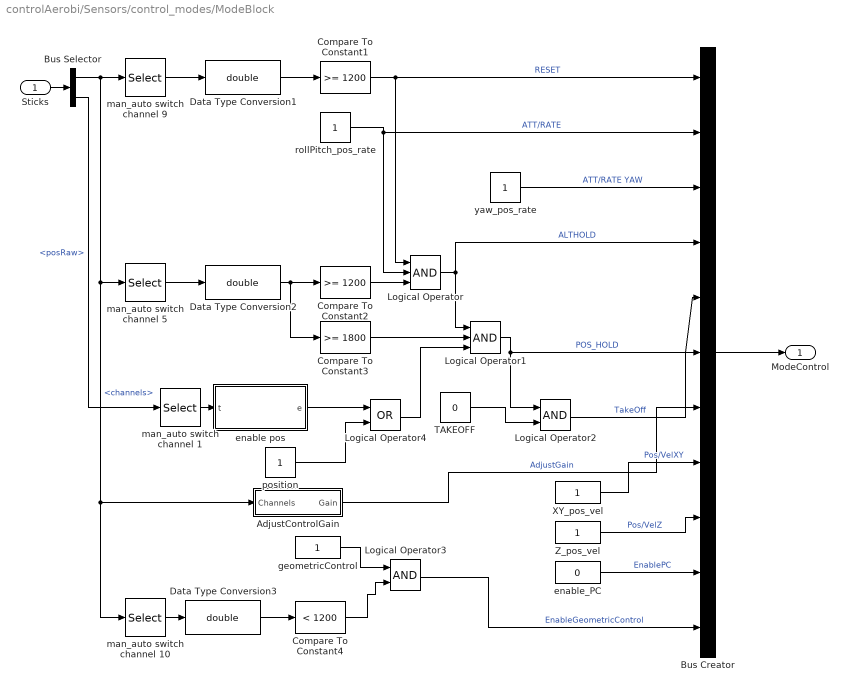
== system controlAerobi/Sensors/control_modes/ModeBlock ==
  Sticks : Inport
  AdjustControlGain : Subsystem
  Bus Creator : BusCreator  Inputs=11
  Bus Selector : BusSelector  OutputSignals=channels,position_.posRaw
  Compare To Constant1 : simulink/Logic and Bit Operations/Compare To Constant  relop=>=  const=1200  OutDataTypeStr=boolean
  Compare To Constant2 : simulink/Logic and Bit Operations/Compare To Constant  relop=>=  const=1200  OutDataTypeStr=boolean
  Compare To Constant3 : simulink/Logic and Bit Operations/Compare To Constant  relop=>=  const=1800  OutDataTypeStr=boolean
  Compare To Constant4 : simulink/Logic and Bit Operations/Compare To Constant  relop=<  const=1200  OutDataTypeStr=boolean
  Data Type Conversion1 : DataTypeConversion  OutDataTypeStr=double
  Data Type Conversion2 : DataTypeConversion  OutDataTypeStr=double
  Data Type Conversion3 : DataTypeConversion  OutDataTypeStr=double
  Logical Operator : Logic  Inputs=3  AllPortsSameDT=off  OutDataTypeStr=boolean
  Logical Operator1 : Logic  Inputs=3  AllPortsSameDT=off  OutDataTypeStr=boolean
  Logical Operator2 : Logic  AllPortsSameDT=off  OutDataTypeStr=boolean
  Logical Operator3 : Logic  AllPortsSameDT=off  OutDataTypeStr=boolean
  Logical Operator4 : Logic  Operator=OR  AllPortsSameDT=off  OutDataTypeStr=boolean
  TAKEOFF : Constant  Value=0  OutDataTypeStr=boolean
  XY_pos_vel : Constant  OutDataTypeStr=boolean
  Z_pos_vel : Constant  OutDataTypeStr=boolean
  enable pos : MATLAB Function  TreatAsAtomicUnit=on
  enable_PC : Constant  Value=0  OutDataTypeStr=boolean
  geometricControl : Constant  OutDataTypeStr=boolean
  man_auto switch channel 1 : Selector  InputPortWidth=5  IndexOptions=Index vector (dialog)  Indices=[5]  OutputSizes=1
  man_auto switch channel 10 : Selector  InputPortWidth=10  IndexOptions=Index vector (dialog)  Indices=[10]  OutputSizes=1
  man_auto switch channel 5 : Selector  InputPortWidth=10  IndexOptions=Index vector (dialog)  Indices=[5]  OutputSizes=1
  man_auto switch channel 9 : Selector  InputPortWidth=10  IndexOptions=Index vector (dialog)  Indices=[8]  OutputSizes=1
  position : Constant  OutDataTypeStr=boolean
  rollPitch_pos_rate : Constant  OutDataTypeStr=boolean
  yaw_pos_rate : Constant  OutDataTypeStr=boolean
  ModeControl : Outport
  wires:
  man_auto switch channel 9/1 -> Data Type Conversion1/1
  Data Type Conversion1/1 -> Compare To Constant1/1
  man_auto switch channel 5/1 -> Data Type Conversion2/1
  Data Type Conversion2/1 -> Compare To Constant2/1, Compare To Constant3/1
  rollPitch_pos_rate/1 -> Logical Operator/2, Bus Creator/2  "ATT/RATE"
  Logical Operator/1 -> Logical Operator1/1, Bus Creator/4  "ALTHOLD"
  Logical Operator1/1 -> Logical Operator2/1, Bus Creator/5  "POS_HOLD"
  Compare To Constant3/1 -> Logical Operator1/2
  Bus Creator/1 -> ModeControl/1
  Sticks/1 -> Bus Selector/1
  Bus Selector/1 -> man_auto switch channel 9/1, man_auto switch channel 10/1, AdjustControlGain/1(Channels), man_auto switch channel 5/1  "<channels>"
  AdjustControlGain/1(Gain) -> Bus Creator/7  "AdjustGain"
  Logical Operator2/1 -> Bus Creator/6  "TakeOff"
  yaw_pos_rate/1 -> Bus Creator/3  "ATT/RATE YAW"
  Compare To Constant1/1 -> Bus Creator/1, Logical Operator/1  "RESET"
  TAKEOFF/1 -> Logical Operator2/2
  Compare To Constant2/1 -> Logical Operator/3
  Bus Selector/2 -> man_auto switch channel 1/1  "<posRaw>"
  man_auto switch channel 1/1 -> enable pos/1(t)
  XY_pos_vel/1 -> Bus Creator/8  "Pos/VelXY"
  Z_pos_vel/1 -> Bus Creator/9  "Pos/VelZ"
  enable_PC/1 -> Bus Creator/10  "EnablePC"
  geometricControl/1 -> Logical Operator3/1
  Logical Operator3/1 -> Bus Creator/11  "EnableGeometricControl"
  man_auto switch channel 10/1 -> Data Type Conversion3/1
  Data Type Conversion3/1 -> Compare To Constant4/1
  Compare To Constant4/1 -> Logical Operator3/2
  enable pos/1(e) -> Logical Operator4/1
  Logical Operator4/1 -> Logical Operator1/3
  position/1 -> Logical Operator4/2

== system controlAerobi/Sensors/control_modes/PositionDesired ==
  Bus Creator : BusCreator  Inputs=4
  Xdes : Constant  Value=0
  YAWdes : Constant  Value=0
  Ydes : Constant  Value=0
  Zdes : Constant
  PositionDesired : Outport
  wires:
  Xdes/1 -> Bus Creator/1  "Xdes"
  Ydes/1 -> Bus Creator/2  "Ydes"
  Zdes/1 -> Bus Creator/3  "Zdes"
  YAWdes/1 -> Bus Creator/4  "YAWdes"
  Bus Creator/1 -> PositionDesired/1

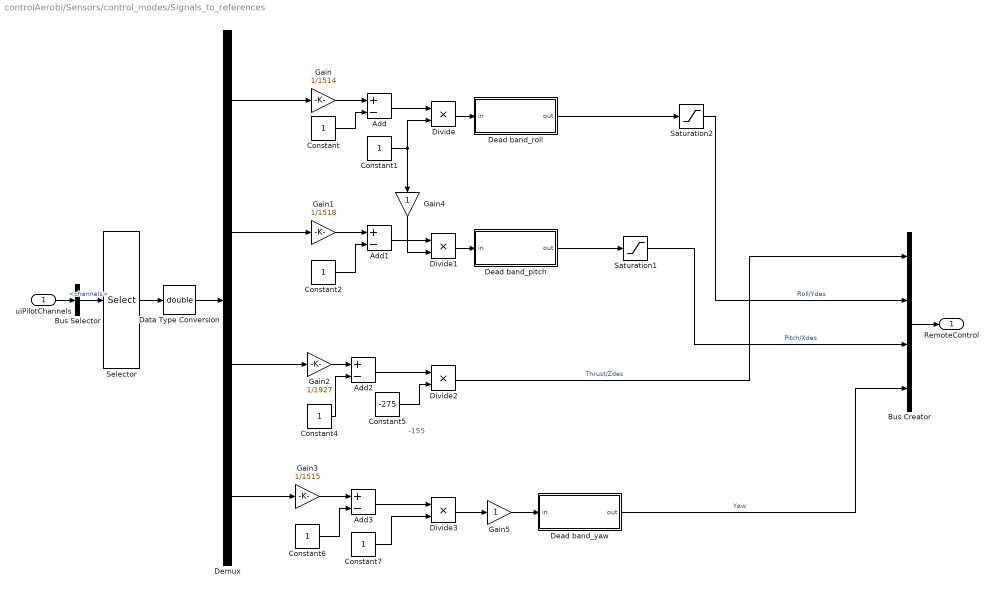
== system controlAerobi/Sensors/control_modes/Signals_to_references ==
  note: -155
  uiPilotChannels : Inport
  Add{,1..3} (4 alike) : Sum  Inputs=+-
  Bus Creator : BusCreator  Inputs=4
  Bus Selector : BusSelector  OutputSignals=channels
  Constant{,1..2,4,6..7} (6 alike) : Constant
  Constant5 : Constant  Value=-275
  Data Type Conversion : DataTypeConversion  OutDataTypeStr=double
  Dead band_pitch : Subsystem
  Dead band_roll : Subsystem
  Dead band_yaw : Subsystem
  Demux : Demux
  Divide{,1..3} (4 alike) : Product  Inputs=**
  Gain : Gain  Gain=1/1514
  Gain1 : Gain  Gain=1/1518
  Gain2 : Gain  Gain=1/1927
  Gain3 : Gain  Gain=1/1515
  Gain4 : Gain
  Gain5 : Gain
  Saturation1 : Saturate
  Saturation2 : Saturate
  Selector : Selector  InputPortWidth=10  IndexOptions=Index vector (dialog)  Indices=[1 2 3 4]  OutputSizes=1
  RemoteControl : Outport
  wires:
  Selector/1 -> Data Type Conversion/1
  Demux/1 -> Gain/1
  Gain/1 -> Add/1
  Add/1 -> Divide/1
  Constant/1 -> Add/2
  Divide/1 -> Dead band_roll/1(in)
  Gain1/1 -> Add1/1
  Add1/1 -> Divide1/1
  Constant2/1 -> Add1/2
  Constant5/1 -> Divide2/2
  Gain3/1 -> Add3/1
  Add3/1 -> Divide3/1
  Constant6/1 -> Add3/2
  Constant7/1 -> Divide3/2
  Demux/4 -> Gain3/1
  Demux/3 -> Gain2/1
  Demux/2 -> Gain1/1
  Divide1/1 -> Dead band_pitch/1(in)
  Divide2/1 -> Bus Creator/1  "Thrust/Zdes"
  Divide3/1 -> Gain5/1
  Data Type Conversion/1 -> Demux/1
  Gain2/1 -> Add2/1
  Add2/1 -> Divide2/1
  Constant4/1 -> Add2/2
  Dead band_roll/1(out) -> Saturation2/1
  Dead band_pitch/1(out) -> Saturation1/1
  Constant1/1 -> Divide/2, Gain4/1
  Gain4/1 -> Divide1/2
  Saturation1/1 -> Bus Creator/3  "Pitch/Xdes"
  Dead band_yaw/1(out) -> Bus Creator/4  "Yaw"
  Saturation2/1 -> Bus Creator/2  "Roll/Ydes"
  Bus Creator/1 -> RemoteControl/1
  uiPilotChannels/1 -> Bus Selector/1
  Bus Selector/1 -> Selector/1  "<channels>"
  Gain5/1 -> Dead band_yaw/1(in)

== system controlAerobi/Sensors/position/EKF_total_Station_Lidar ==
  I_totalStation : Inport  OutDataTypeStr=Bus: shm_totalStation
  I_sf11c : Inport  Port=2  OutDataTypeStr=Bus: shm_lightware
  attitude_ : Inport  Port=3
  d_sf11 : Inport  Port=4
  d_prism : Inport  Port=5
  KQ : Inport  Port=6
  KR : Inport  Port=7
  ControlModes : Inport  Port=8
  Acc : BusToVector
  Bus Selector : BusSelector  OutputSignals=_z
  Bus Selector1 : BusSelector  OutputSignals=AngularPosition.roll,AngularPosition.pitch,AngularPosition.yaw,Accelerometer
  Bus Selector3 : BusSelector  OutputSignals=RemoteControl.Thrust/Zdes
  Data Type Conversion : DataTypeConversion  OutDataTypeStr=double
  Mux : Mux  Inputs=2
  Mux1 : Mux  Inputs=3
  Mux2 : Mux  Inputs=3
  enu/ned : Subsystem
  filter : Subsystem
  routingData : Subsystem
  NED_position : Outport
  NED_speed : Outport  Port=2
  posRaw : Outport  Port=3
  wires:
  Mux/1 -> posRaw/1  "posRaw"
  attitude_/1 -> Bus Selector1/1
  Data Type Conversion/1 -> Mux/1, filter/4(z)
  Bus Selector/1 -> Data Type Conversion/1  "<_z>"
  Bus Selector1/4 -> Acc/1  "<Accelerometer>"
  Bus Selector1/3 -> filter/7(yaw)  "<yaw>"
  I_sf11c/1 -> Bus Selector/1
  Mux2/1 -> NED_speed/1
  Mux1/1 -> NED_position/1
  Bus Selector1/1 -> filter/5(roll)  "<roll>"
  Bus Selector1/2 -> filter/6(pitch)  "<pitch>"
  Acc/1 -> filter/8(a_b)
  d_sf11/1 -> filter/9(d_sf11)
  d_prism/1 -> filter/10(d_prism)
  KQ/1 -> filter/11(KQ)
  KR/1 -> filter/12(KR)
  filter/1(x_hat) -> Mux1/1  "x"
  filter/2(y_hat) -> Mux1/2  "y"
  filter/3(z_hat) -> Mux1/3  "z"
  filter/4(dx_hat) -> Mux2/1  "dx"
  filter/5(dy_hat) -> Mux2/2  "dy"
  filter/6(dz_hat) -> Mux2/3  "dz"
  ControlModes/1 -> Bus Selector3/1
  Bus Selector3/1 -> filter/13(thrust)  "<Thrust/Zdes>"
  I_totalStation/1 -> routingData/1(I_totalStation), enu/ned/1(I_totalStation)
  enu/ned/1(timeTS) -> filter/1(timeTS)
  enu/ned/2(x) -> filter/2(x)
  enu/ned/3(y) -> filter/3(y)
  routingData/1(totalStation) -> Mux/2

== system controlAerobi/Sensors/position/GPS_px4 ==
  I_localPositionPX4EKF2 : Inport  OutDataTypeStr=Bus: shm_localPositionPX4EKF2
  NED estimation : Subsystem
  Zero-Order Hold2 : ZeroOrderHold  SampleTime=Ts
  Zero-Order Hold4 : ZeroOrderHold  SampleTime=Ts
  NED_position : Outport
  NED_speed : Outport  Port=2
  wires:
  NED estimation/1(NED position) -> Zero-Order Hold2/1
  NED estimation/2(NED speed) -> Zero-Order Hold4/1
  Zero-Order Hold2/1 -> NED_position/1
  Zero-Order Hold4/1 -> NED_speed/1
  I_localPositionPX4EKF2/1 -> NED estimation/1(I_localPositionPX4EKF2)

== system controlAerobi/Sensors/position/px4fow ==
  attitude_ : Inport
  ControlModes : Inport  Port=2
  I_px4flow : Inport  Port=3  OutDataTypeStr=Bus: shm_px4flow
  Acc : BusToVector
  Bus Creator : BusCreator  Inputs=4
  Bus Selector : BusSelector  OutputSignals=_velocity_x,_velocity_y,_ground_distance,_quality
  Bus Selector1 : BusSelector  OutputSignals=dx,dy,quality
  Bus Selector2 : BusSelector  OutputSignals=AngularPosition.roll,AngularPosition.pitch,AngularPosition.yaw,Accelerometer
  Bus Selector3 : BusSelector  OutputSignals=RemoteControl.Thrust/Zdes
  Data Type Conversion{,1..2,5} (4 alike) : DataTypeConversion  OutDataTypeStr=double
  Gain : Gain  Gain=0.001
  Gain1 : Gain  Gain=0.001
  Gain2 : Gain
  Gain3 : Gain  Gain=1/255
  Gain4 : Gain  Gain=0
  Gain5 : Gain  Gain=0.001
  Liner Fixed-gain Filter1 : MATLAB Function  TreatAsAtomicUnit=on
  Mux : Mux  Inputs=5
  dxdyaxay : Outport
  wires:
  I_px4flow/1 -> Bus Selector/1
  Data Type Conversion/1 -> Gain/1
  Data Type Conversion1/1 -> Gain1/1
  Bus Selector/1 -> Data Type Conversion/1  "<_velocity_x>"
  Bus Selector/2 -> Data Type Conversion1/1  "<_velocity_y>"
  Data Type Conversion5/1 -> Gain5/1
  Bus Selector/3 -> Data Type Conversion5/1  "<_ground_distance>"
  Data Type Conversion2/1 -> Gain2/1
  Bus Selector/4 -> Data Type Conversion2/1  "<_quality>"
  Gain5/1 -> Bus Creator/3  "z"
  Gain2/1 -> Gain3/1, Bus Creator/4  "quality"
  Bus Creator/1 -> Bus Selector1/1
  Gain/1 -> Bus Creator/2  "dy"
  Gain1/1 -> Bus Creator/1  "dx"
  ControlModes/1 -> Bus Selector3/1
  Bus Selector3/1 -> Liner Fixed-gain Filter1/1(thrust)  "<Thrust/Zdes>"
  Bus Selector1/2 -> Liner Fixed-gain Filter1/3(dy)  "<dy>"
  Bus Selector1/1 -> Liner Fixed-gain Filter1/2(dx)  "<dx>"
  Bus Selector1/3 -> Liner Fixed-gain Filter1/4(quality)  "<quality>"
  Bus Selector2/4 -> Acc/1  "<Accelerometer>"
  attitude_/1 -> Bus Selector2/1
  Bus Selector2/3 -> Gain4/1  "<yaw>"
  Bus Selector2/2 -> Liner Fixed-gain Filter1/6(pitch)  "<pitch>"
  Bus Selector2/1 -> Liner Fixed-gain Filter1/5(roll)  "<roll>"
  Acc/1 -> Liner Fixed-gain Filter1/8(a_b)
  Mux/1 -> dxdyaxay/1
  Liner Fixed-gain Filter1/1(vx) -> Mux/1
  Liner Fixed-gain Filter1/2(vy) -> Mux/2
  Liner Fixed-gain Filter1/3(ax) -> Mux/3
  Liner Fixed-gain Filter1/4(ay) -> Mux/4
  Gain3/1 -> Mux/5
  Gain4/1 -> Liner Fixed-gain Filter1/7(yaw)

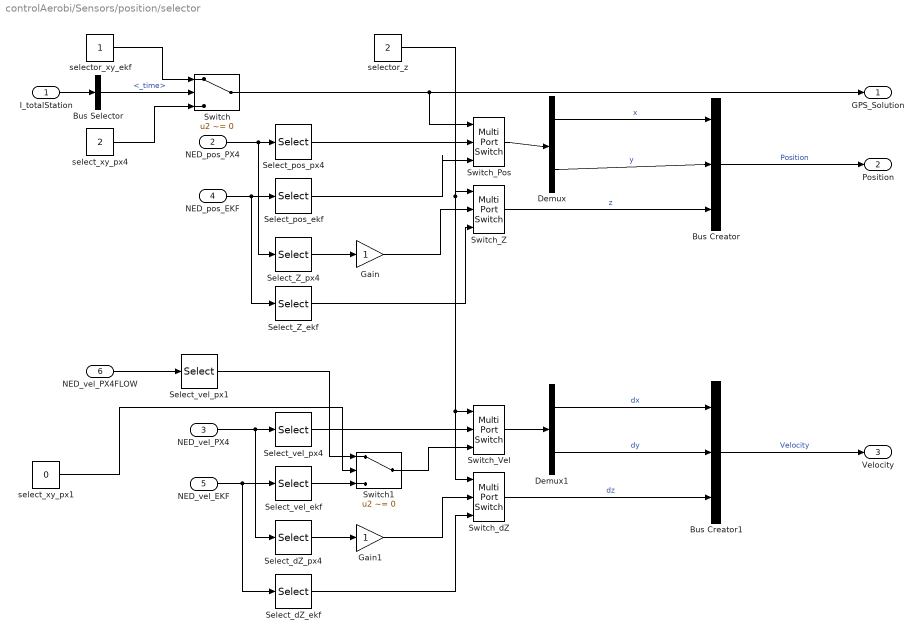
== system controlAerobi/Sensors/position/selector ==
  I_totalStation : Inport  OutDataTypeStr=Bus: shm_totalStation
  NED_pos_PX4 : Inport  Port=2
  NED_vel_PX4 : Inport  Port=3
  NED_pos_EKF : Inport  Port=4
  NED_vel_EKF : Inport  Port=5
  NED_vel_PX4FLOW : Inport  Port=6
  Bus Creator : BusCreator  Inputs=3
  Bus Creator1 : BusCreator  Inputs=3
  Bus Selector : BusSelector  OutputSignals=_time
  Demux : Demux  Outputs=2
  Demux1 : Demux  Outputs=2
  Gain : Gain
  Gain1 : Gain
  Select_Z_ekf : Selector  InputPortWidth=3  IndexOptions=Index vector (dialog)  Indices=[3]  OutputSizes=1
  Select_Z_px4 : Selector  InputPortWidth=3  IndexOptions=Index vector (dialog)  Indices=[3]  OutputSizes=1
  Select_dZ_ekf : Selector  InputPortWidth=3  IndexOptions=Index vector (dialog)  Indices=[3]  OutputSizes=1
  Select_dZ_px4 : Selector  InputPortWidth=3  IndexOptions=Index vector (dialog)  Indices=[3]  OutputSizes=1
  Select_pos_ekf : Selector  InputPortWidth=3  IndexOptions=Index vector (dialog)  Indices=[1 2]  OutputSizes=1
  Select_pos_px4 : Selector  InputPortWidth=3  IndexOptions=Index vector (dialog)  Indices=[1 2]  OutputSizes=1
  Select_vel_ekf : Selector  InputPortWidth=3  IndexOptions=Index vector (dialog)  Indices=[1 2]  OutputSizes=1
  Select_vel_px1 : Selector  InputPortWidth=5  IndexOptions=Index vector (dialog)  Indices=[1 2]  OutputSizes=1
  Select_vel_px4 : Selector  InputPortWidth=3  IndexOptions=Index vector (dialog)  Indices=[1 2]  OutputSizes=1
  Switch : Switch  Criteria=u2 ~= 0
  Switch1 : Switch  Criteria=u2 ~= 0
  Switch_Pos : MultiPortSwitch  Inputs=2
  Switch_Vel : MultiPortSwitch  Inputs=2
  Switch_Z : MultiPortSwitch  Inputs=2
  Switch_dZ : MultiPortSwitch  Inputs=2
  select_xy_px1 : Constant  Value=0
  select_xy_px4 : Constant  Value=2
  selector_xy_ekf : Constant
  selector_z : Constant  Value=2
  GPS_Solution : Outport
  Position : Outport  Port=2
  Velocity : Outport  Port=3
  wires:
  Bus Creator/1 -> Position/1  "Position"
  Bus Creator1/1 -> Velocity/1  "Velocity"
  Switch_Pos/1 -> Demux/1
  Demux/1 -> Bus Creator/1  "x"
  Demux/2 -> Bus Creator/2  "y"
  Switch_Vel/1 -> Demux1/1
  Demux1/2 -> Bus Creator1/2  "dy"
  Demux1/1 -> Bus Creator1/1  "dx"
  Switch/1 -> GPS_Solution/1, Switch_Pos/1
  Switch_Z/1 -> Bus Creator/3  "z"
  NED_pos_PX4/1 -> Select_Z_px4/1, Select_pos_px4/1
  Select_pos_px4/1 -> Switch_Pos/2
  NED_pos_EKF/1 -> Select_Z_ekf/1, Select_pos_ekf/1
  Select_pos_ekf/1 -> Switch_Pos/3
  Select_vel_px4/1 -> Switch_Vel/2
  selector_z/1 -> Switch_Vel/1, Switch_dZ/1, Switch_Z/1
  Select_Z_px4/1 -> Gain/1
  Select_Z_ekf/1 -> Switch_Z/3
  Switch_dZ/1 -> Bus Creator1/3  "dz"
  NED_vel_PX4/1 -> Select_dZ_px4/1, Select_vel_px4/1
  NED_vel_EKF/1 -> Select_dZ_ekf/1, Select_vel_ekf/1
  Select_dZ_px4/1 -> Gain1/1
  Select_dZ_ekf/1 -> Switch_dZ/3
  I_totalStation/1 -> Bus Selector/1
  Bus Selector/1 -> Switch/2  "<_time>"
  selector_xy_ekf/1 -> Switch/1
  select_xy_px4/1 -> Switch/3
  Gain/1 -> Switch_Z/2
  Gain1/1 -> Switch_dZ/2
  Select_vel_ekf/1 -> Switch1/3
  Switch1/1 -> Switch_Vel/3
  NED_vel_PX4FLOW/1 -> Select_vel_px1/1
  select_xy_px1/1 -> Switch1/2
  Select_vel_px1/1 -> Switch1/1

== system controlAerobi/Sensors/position/svo ==
  I_svo : Inport  OutDataTypeStr=Bus: shm_svo
  Bus Selector : BusSelector  OutputSignals=_x,_y,_z,_qx,_qy,_qz,_qw
  Mux : Mux  Inputs=7
  Select XYZ : Selector  InputPortWidth=7  IndexOptions=Index vector (dialog)  Indices=[1 2 3]  OutputSizes=1
  XYZ : Outport
  wires:
  Select XYZ/1 -> XYZ/1
  I_svo/1 -> Bus Selector/1
  Bus Selector/1 -> Mux/1  "<_x>"
  Bus Selector/2 -> Mux/2  "<_y>"
  Bus Selector/3 -> Mux/3  "<_z>"
  Bus Selector/4 -> Mux/4  "<_qx>"
  Bus Selector/5 -> Mux/5  "<_qy>"
  Bus Selector/6 -> Mux/6  "<_qz>"
  Bus Selector/7 -> Mux/7  "<_qw>"
  Mux/1 -> Select XYZ/1
